simulink model "cranesimu"  (R2015a)
settings: Solver=ode45  StartTime=0.0  StopTime=20.0  RelTol=1e-3
libraries: cstblocks x3, simulink x1
settings Model: Creator=roevhat  LastModifiedBy=morten

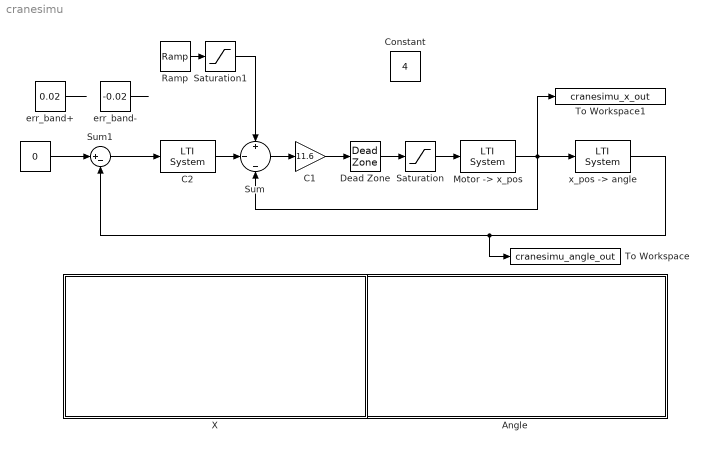
== system cranesimu ==
  " " : Constant  Value=0
  " err_band+" : Constant  Value=0.02
  " err_band-" : Constant  Value=-0.02
  Angle : Subsystem  DialogController=hmiCreateDDGDialog  IsWebBlock=on  mask(MathWorksWebBlock){webBlockId=a8e75964-e3a8-414a-b4cf-d80626da48bf, webBlockType=sdiscope, ShowInitialText=on, HMISrcModelName=cranesimu}
      mask prompts: webBlockId "WebBlock Id"; webBlockType "WebBlock Type"; HMISrcModelName "Source Model"
      mask Help: helpview([docroot '/mapfiles/simulink.map'], 'hmi_scope')
      mask Display:
      | if strcmp(get_param(bdroot(gcb),'BlockDiagramType'), 'library')
      |     image([(matlabroot) '/toolbox/simulink/hmi/icons/DashboardScope.png']);
      | end
  C1 : Gain  Gain=11.6
  C2 : cstblocks/LTI System  sys=C2  IC=[]
  Constant : Constant  Value=4
  Dead Zone : DeadZone  LowerValue=-5  UpperValue=5  SaturateOnIntegerOverflow=on
  "Motor -> x_pos" : cstblocks/LTI System  sys=X  IC=[]
  Ramp : simulink/Sources/Ramp  slope=.5  start=0  X0=0
  Saturation : Saturate  UpperLimit=14  LowerLimit=-14
  Saturation1 : Saturate  UpperLimit=4  LowerLimit=0
  Sum : Sum  Inputs=+|-|-
  Sum1 : Sum  Inputs=|+-
  To Workspace : ToWorkspace  VariableName=cranesimu_angle_out  SaveFormat=Timeseries  SampleTime=-1
  To Workspace1 : ToWorkspace  VariableName=cranesimu_x_out  SaveFormat=Timeseries  SampleTime=-1
  X : Subsystem  DialogController=hmiCreateDDGDialog  IsWebBlock=on  mask(MathWorksWebBlock){webBlockId=2ac42065-2a1d-45d8-b9d1-76f78bc34ac1, webBlockType=sdiscope, ShowInitialText=on, HMISrcModelName=cranesimu}
      mask prompts: webBlockId "WebBlock Id"; webBlockType "WebBlock Type"; HMISrcModelName "Source Model"
      mask Help: helpview([docroot '/mapfiles/simulink.map'], 'hmi_scope')
      mask Display:
      | if strcmp(get_param(bdroot(gcb),'BlockDiagramType'), 'library')
      |     image([(matlabroot) '/toolbox/simulink/hmi/icons/DashboardScope.png']);
      | end
  "x_pos -> angle" : cstblocks/LTI System  sys=W  IC=[]
  wires:
  "Motor -> x_pos"/1 -> To Workspace1/1, "x_pos -> angle"/1, Sum/3
  "x_pos -> angle"/1 -> To Workspace/1, Sum1/2
  Sum/1 -> C1/1
  " "/1 -> Sum1/1
  Ramp/1 -> Saturation1/1
  Sum1/1 -> C2/1
  C1/1 -> Dead Zone/1
  Saturation/1 -> "Motor -> x_pos"/1
  C2/1 -> Sum/2
  " err_band+"/1 -> ?
  " err_band-"/1 -> ?
  Dead Zone/1 -> Saturation/1
  Saturation1/1 -> Sum/1

== system cranesimu/Angle ==

== system cranesimu/X ==
